simulink subsystem "heading_generator"  (R2023a)
settings: Solver=VariableStepAuto  StartTime=0.0  StopTime=10.0  RelTol=1e-3
libraries: simulink x2, eeGeneralControl x1
settings Model: Creator=thesa  LastModifiedBy=thesa

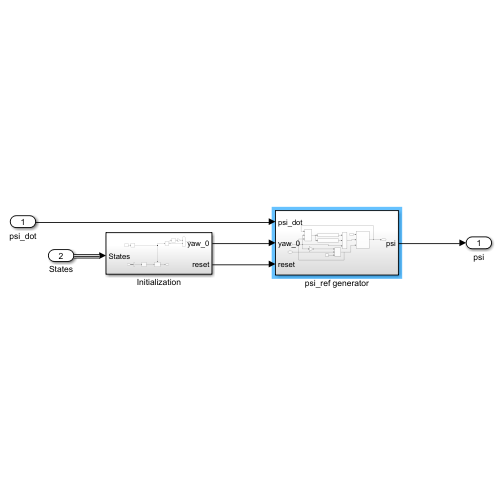
[thumbnail: Simulink's stored preview of the top-level diagram]
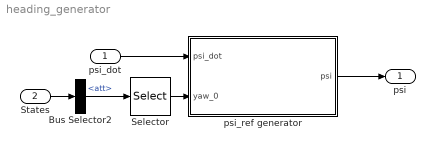
== system heading_generator ==
  psi_dot : Inport
  States : Inport  Port=2
  Bus Selector2 : BusSelector  OutputSignals=att
  Selector : Selector  InputPortWidth=3  IndexOptions=Index vector (dialog)  Indices=[3]  OutputSizes=1
  psi_ref generator : Subsystem
  psi : Outport
  wires:
  psi_ref generator/1(psi) -> psi/1
  psi_dot/1 -> psi_ref generator/1(psi_dot)
  Selector/1 -> psi_ref generator/2(yaw_0)
  Bus Selector2/1 -> Selector/1  "<att>"
  States/1 -> Bus Selector2/1

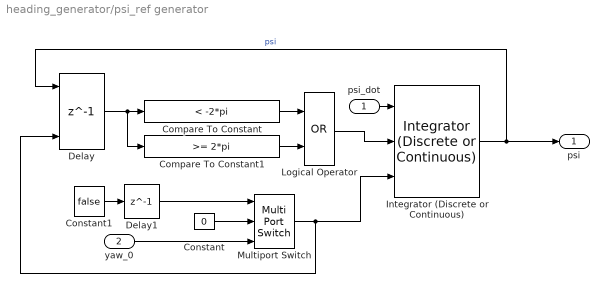
== system heading_generator/psi_ref generator ==
  psi_dot : Inport
  yaw_0 : Inport  Port=2
  Compare To Constant : simulink/Logic and Bit Operations/Compare To Constant  relop=<  const=-2*pi  OutDataTypeStr=boolean
  Compare To Constant1 : simulink/Logic and Bit Operations/Compare To Constant  relop=>=  const=2*pi  OutDataTypeStr=boolean
  Constant : Constant  Value=0
  Constant1 : Constant  Value=false
  Delay : Delay  DelayLength=1  InitialConditionSource=Input port  ExternalReset=Rising
      settings: InputPortMap=u0,r5,p4
  Delay1 : Delay  DelayLength=1  InitialCondition=true
  Integrator (Discrete or Continuous) : eeGeneralControl/Integrator (Discrete or Continuous)  LabelModeActiveChoice=Discrete  ExternalReset=rising  LimitType=Windup  B=inf  A=-inf  Ts=-1
      settings: LibrarySourceBlock=|
      | ee_sl_lib/General Control/Integrator
      | (Discrete or Continuous)
  Logical Operator : Logic  Operator=OR  AllPortsSameDT=off  OutDataTypeStr=boolean
  Multiport Switch : MultiPortSwitch  DataPortOrder=Zero-based contiguous  Inputs=2  DiagnosticForDefault=None  zeroidx=on  SaturateOnIntegerOverflow=off  InputSameDT=off
  psi : Outport
  wires:
  Constant1/1 -> Delay1/1
  Multiport Switch/1 -> Integrator (Discrete or Continuous)/3, Delay/3
  Delay1/1 -> Multiport Switch/1
  Constant/1 -> Multiport Switch/2
  Delay/1 -> Compare To Constant/1, Compare To Constant1/1
  yaw_0/1 -> Multiport Switch/3
  Compare To Constant/1 -> Logical Operator/1
  Compare To Constant1/1 -> Logical Operator/2
  Logical Operator/1 -> Integrator (Discrete or Continuous)/2
  psi_dot/1 -> Integrator (Discrete or Continuous)/1
  Integrator (Discrete or Continuous)/1 -> psi/1, Delay/1  "psi"
